simulink library "MultiBodyLibrary"  (R2021b)
settings: Solver=VariableStepAuto  StartTime=0.0  StopTime=10.0  RelTol=1e-3
undefined symbols (not defined in the file or in its folder): gainStruct, useConstraint
libraries: RobotStateLibrary x23, $bdroot x1
settings Model: Creator=icub  LastModifiedBy=icub
settings SolverCC: AlgebraicLoopSolver=TrustRegion
settings DebuggingCC: SFMachineParentedDataDiag=warning

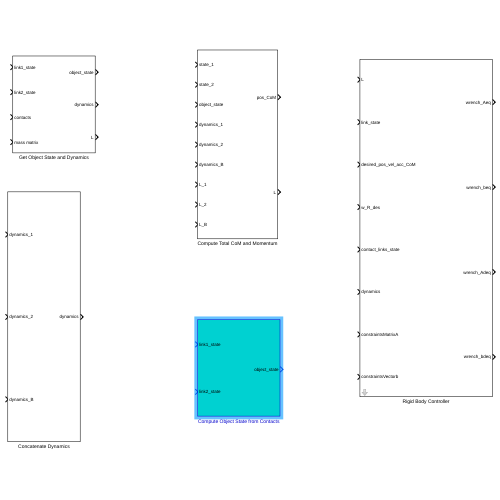
[thumbnail: Simulink's stored preview of the top-level diagram]
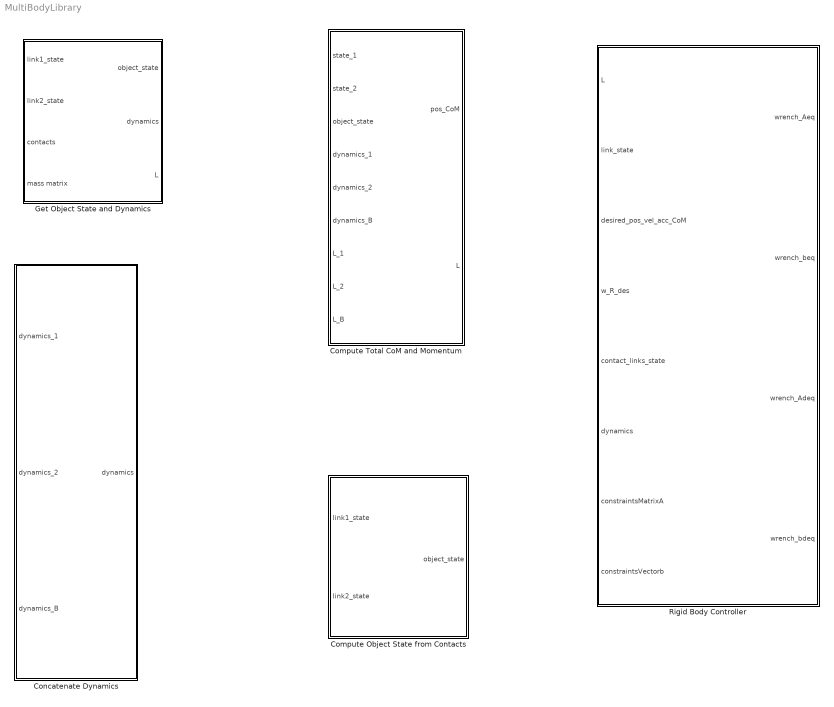
== system MultiBodyLibrary ==
  Compute Object State from Contacts : Subsystem
  Compute Total CoM and Momentum : Subsystem
  Concatenate Dynamics : Subsystem
  Get Object State and Dynamics : Subsystem
  Rigid Body Controller : Subsystem  mask{GainMomentum=gainStruct, linksUseConstraintMatrix=useConstraint}
      mask prompts: GainMomentum "Momentum Control Gain"; linksUseConstraintMatrix "Use Force Constraint on Links"

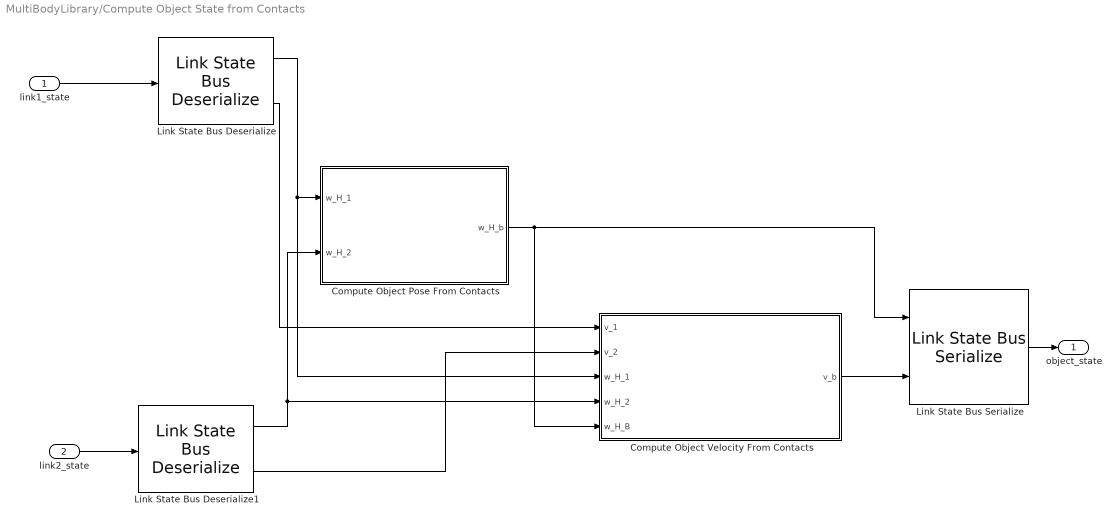
== system MultiBodyLibrary/Compute Object State from Contacts ==
  link1_state : Inport
  link2_state : Inport  Port=2
  Compute Object Pose From Contacts : Subsystem
  Compute Object Velocity From Contacts : Subsystem
  Link State Bus Deserialize : RobotStateLibrary/Link State Bus Deserialize  SystemSampleTime=-1  VariantActivationTime=update diagram  Latency=0  AutoFrameSizeCalculation=off
      settings: SourceProductName=robot-state-library
  Link State Bus Deserialize1 : RobotStateLibrary/Link State Bus Deserialize  SystemSampleTime=-1  VariantActivationTime=update diagram  Latency=0  AutoFrameSizeCalculation=off
      settings: SourceProductName=robot-state-library
  Link State Bus Serialize : RobotStateLibrary/Link State Bus Serialize  SystemSampleTime=-1  VariantActivationTime=update diagram  Latency=0  AutoFrameSizeCalculation=off
      settings: SourceProductName=robot-state-library
  object_state : Outport
  wires:
  Link State Bus Deserialize/1 -> Compute Object Velocity From Contacts/3(w_H_1), Compute Object Pose From Contacts/1(w_H_1)
  Link State Bus Deserialize/2 -> Compute Object Velocity From Contacts/1(v_1)
  Link State Bus Deserialize1/2 -> Compute Object Velocity From Contacts/2(v_2)
  Link State Bus Deserialize1/1 -> Compute Object Velocity From Contacts/4(w_H_2), Compute Object Pose From Contacts/2(w_H_2)
  Compute Object Pose From Contacts/1(w_H_b) -> Link State Bus Serialize/1, Compute Object Velocity From Contacts/5(w_H_B)
  link1_state/1 -> Link State Bus Deserialize/1
  link2_state/1 -> Link State Bus Deserialize1/1
  Compute Object Velocity From Contacts/1(v_b) -> Link State Bus Serialize/2
  Link State Bus Serialize/1 -> object_state/1

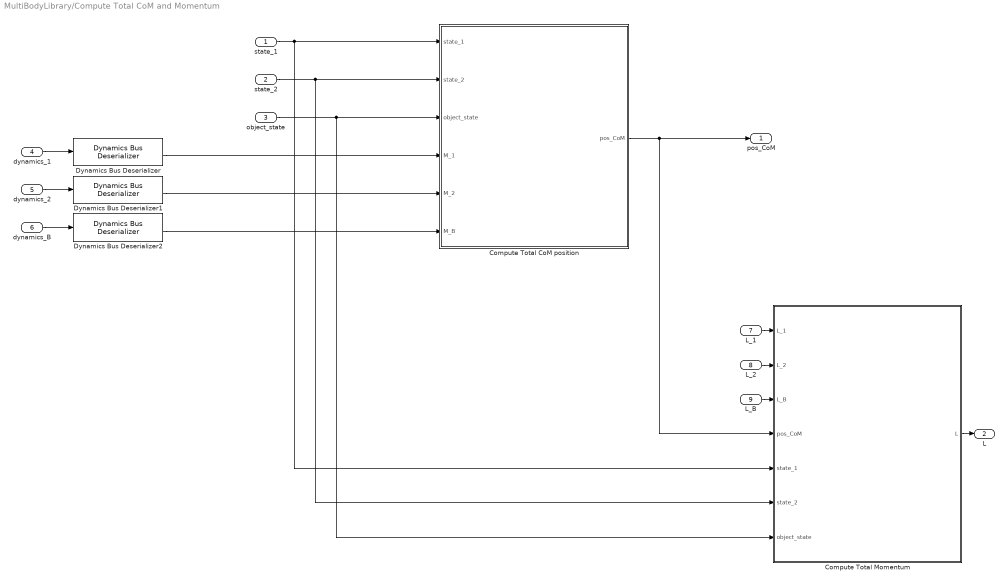
== system MultiBodyLibrary/Compute Total CoM and Momentum ==
  state_1 : Inport
  state_2 : Inport  Port=2
  object_state : Inport  Port=3
  dynamics_1 : Inport  Port=4
  dynamics_2 : Inport  Port=5
  dynamics_B : Inport  Port=6
  L_1 : Inport  Port=7
  L_2 : Inport  Port=8
  L_B : Inport  Port=9
  Compute Total CoM position : Subsystem
  Compute Total Momentum : Subsystem
  Dynamics Bus Deserializer : RobotStateLibrary/Dynamics Bus Deserializer  SystemSampleTime=-1  VariantActivationTime=update diagram  Latency=0  AutoFrameSizeCalculation=off
      settings: SourceProductName=robot-state-library
  Dynamics Bus Deserializer1 : RobotStateLibrary/Dynamics Bus Deserializer  SystemSampleTime=-1  VariantActivationTime=update diagram  Latency=0  AutoFrameSizeCalculation=off
      settings: SourceProductName=robot-state-library
  Dynamics Bus Deserializer2 : RobotStateLibrary/Dynamics Bus Deserializer  SystemSampleTime=-1  VariantActivationTime=update diagram  Latency=0  AutoFrameSizeCalculation=off
      settings: SourceProductName=robot-state-library
  pos_CoM : Outport
  L : Outport  Port=2
  wires:
  L_B/1 -> Compute Total Momentum/3(L_B)
  L_2/1 -> Compute Total Momentum/2(L_2)
  object_state/1 -> Compute Total Momentum/7(object_state), Compute Total CoM position/3(object_state)
  L_1/1 -> Compute Total Momentum/1(L_1)
  Compute Total CoM position/1(pos_CoM) -> Compute Total Momentum/4(pos_CoM), pos_CoM/1
  state_1/1 -> Compute Total Momentum/5(state_1), Compute Total CoM position/1(state_1)
  Compute Total Momentum/1(L) -> L/1
  state_2/1 -> Compute Total Momentum/6(state_2), Compute Total CoM position/2(state_2)
  Dynamics Bus Deserializer/3 -> Compute Total CoM position/4(M_1)
  dynamics_1/1 -> Dynamics Bus Deserializer/1
  dynamics_2/1 -> Dynamics Bus Deserializer1/1
  Dynamics Bus Deserializer1/3 -> Compute Total CoM position/5(M_2)
  Dynamics Bus Deserializer2/3 -> Compute Total CoM position/6(M_B)
  dynamics_B/1 -> Dynamics Bus Deserializer2/1

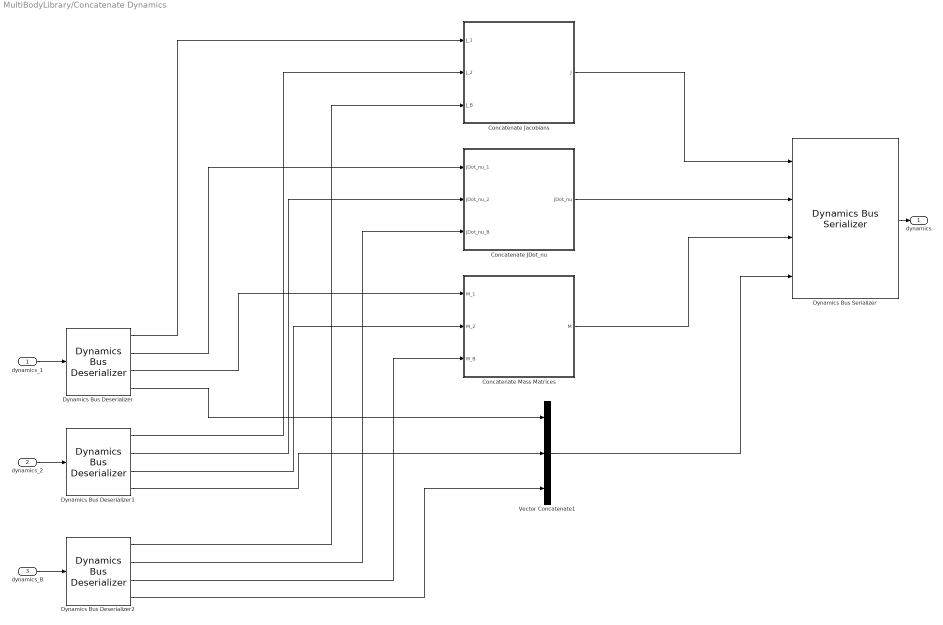
== system MultiBodyLibrary/Concatenate Dynamics ==
  dynamics_1 : Inport
  dynamics_2 : Inport  Port=2
  dynamics_B : Inport  Port=3
  Concatenate JDot_nu : MATLAB Function  TreatAsAtomicUnit=on
  Concatenate Jacobians : MATLAB Function  TreatAsAtomicUnit=on
  Concatenate Mass Matrices : MATLAB Function  TreatAsAtomicUnit=on
  Dynamics Bus Deserializer : RobotStateLibrary/Dynamics Bus Deserializer  SystemSampleTime=-1  VariantActivationTime=update diagram  Latency=0  AutoFrameSizeCalculation=off
      settings: SourceProductName=robot-state-library
  Dynamics Bus Deserializer1 : RobotStateLibrary/Dynamics Bus Deserializer  SystemSampleTime=-1  VariantActivationTime=update diagram  Latency=0  AutoFrameSizeCalculation=off
      settings: SourceProductName=robot-state-library
  Dynamics Bus Deserializer2 : RobotStateLibrary/Dynamics Bus Deserializer  SystemSampleTime=-1  VariantActivationTime=update diagram  Latency=0  AutoFrameSizeCalculation=off
      settings: SourceProductName=robot-state-library
  Dynamics Bus Serializer : RobotStateLibrary/Dynamics Bus Serializer  SystemSampleTime=-1  VariantActivationTime=update diagram  Latency=0  AutoFrameSizeCalculation=off
      settings: SourceProductName=robot-state-library
  Vector Concatenate1 : Concatenate  NumInputs=3
  dynamics : Outport
  wires:
  Dynamics Bus Serializer/1 -> dynamics/1
  Dynamics Bus Deserializer2/4 -> Vector Concatenate1/3
  Concatenate Mass Matrices/1(M) -> Dynamics Bus Serializer/3
  Concatenate Jacobians/1(J) -> Dynamics Bus Serializer/1
  Dynamics Bus Deserializer1/4 -> Vector Concatenate1/2
  Vector Concatenate1/1 -> Dynamics Bus Serializer/4
  Concatenate JDot_nu/1(JDot_nu) -> Dynamics Bus Serializer/2
  Dynamics Bus Deserializer/4 -> Vector Concatenate1/1
  dynamics_1/1 -> Dynamics Bus Deserializer/1
  dynamics_2/1 -> Dynamics Bus Deserializer1/1
  dynamics_B/1 -> Dynamics Bus Deserializer2/1
  Dynamics Bus Deserializer/1 -> Concatenate Jacobians/1(J_1)
  Dynamics Bus Deserializer1/1 -> Concatenate Jacobians/2(J_2)
  Dynamics Bus Deserializer2/1 -> Concatenate Jacobians/3(J_B)
  Dynamics Bus Deserializer/2 -> Concatenate JDot_nu/1(JDot_nu_1)
  Dynamics Bus Deserializer1/2 -> Concatenate JDot_nu/2(JDot_nu_2)
  Dynamics Bus Deserializer2/2 -> Concatenate JDot_nu/3(JDot_nu_B)
  Dynamics Bus Deserializer/3 -> Concatenate Mass Matrices/1(M_1)
  Dynamics Bus Deserializer1/3 -> Concatenate Mass Matrices/2(M_2)
  Dynamics Bus Deserializer2/3 -> Concatenate Mass Matrices/3(M_B)

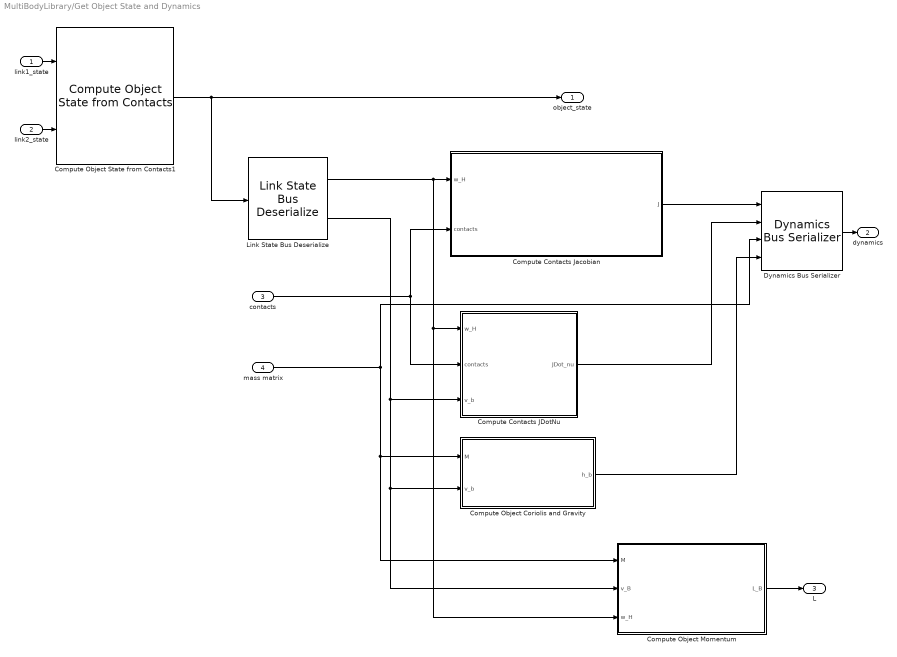
== system MultiBodyLibrary/Get Object State and Dynamics ==
  link1_state : Inport
  link2_state : Inport  Port=2
  contacts : Inport  Port=3
  mass matrix : Inport  Port=4
  Compute Contacts JDotNu : MATLAB Function  TreatAsAtomicUnit=on
  Compute Contacts Jacobian : MATLAB Function  TreatAsAtomicUnit=on
  Compute Object Coriolis and Gravity : MATLAB Function  TreatAsAtomicUnit=on
  Compute Object Momentum : MATLAB Function  TreatAsAtomicUnit=on
  Compute Object State from Contacts1 : $bdroot/Compute Object State from Contacts  SystemSampleTime=-1  VariantActivationTime=update diagram  Latency=0  AutoFrameSizeCalculation=off
  Dynamics Bus Serializer : RobotStateLibrary/Dynamics Bus Serializer  SystemSampleTime=-1  VariantActivationTime=update diagram  Latency=0  AutoFrameSizeCalculation=off
      settings: SourceProductName=robot-state-library
  Link State Bus Deserialize : RobotStateLibrary/Link State Bus Deserialize  SystemSampleTime=-1  VariantActivationTime=update diagram  Latency=0  AutoFrameSizeCalculation=off
      settings: SourceProductName=robot-state-library
  object_state : Outport
  dynamics : Outport  Port=2
  L : Outport  Port=3
  wires:
  link2_state/1 -> Compute Object State from Contacts1/2
  Compute Object State from Contacts1/1 -> Link State Bus Deserialize/1, object_state/1
  link1_state/1 -> Compute Object State from Contacts1/1
  contacts/1 -> Compute Contacts JDotNu/2(contacts), Compute Contacts Jacobian/2(contacts)
  mass matrix/1 -> Compute Object Momentum/1(M), Compute Object Coriolis and Gravity/1(M), Dynamics Bus Serializer/3
  Link State Bus Deserialize/1 -> Compute Object Momentum/3(w_H), Compute Contacts JDotNu/1(w_H), Compute Contacts Jacobian/1(w_H)
  Link State Bus Deserialize/2 -> Compute Object Momentum/2(v_B), Compute Object Coriolis and Gravity/2(v_b), Compute Contacts JDotNu/3(v_b)
  Compute Contacts Jacobian/1(J) -> Dynamics Bus Serializer/1
  Compute Contacts JDotNu/1(JDot_nu) -> Dynamics Bus Serializer/2
  Compute Object Coriolis and Gravity/1(h_b) -> Dynamics Bus Serializer/4
  Dynamics Bus Serializer/1 -> dynamics/1
  Compute Object Momentum/1(L_B) -> L/1

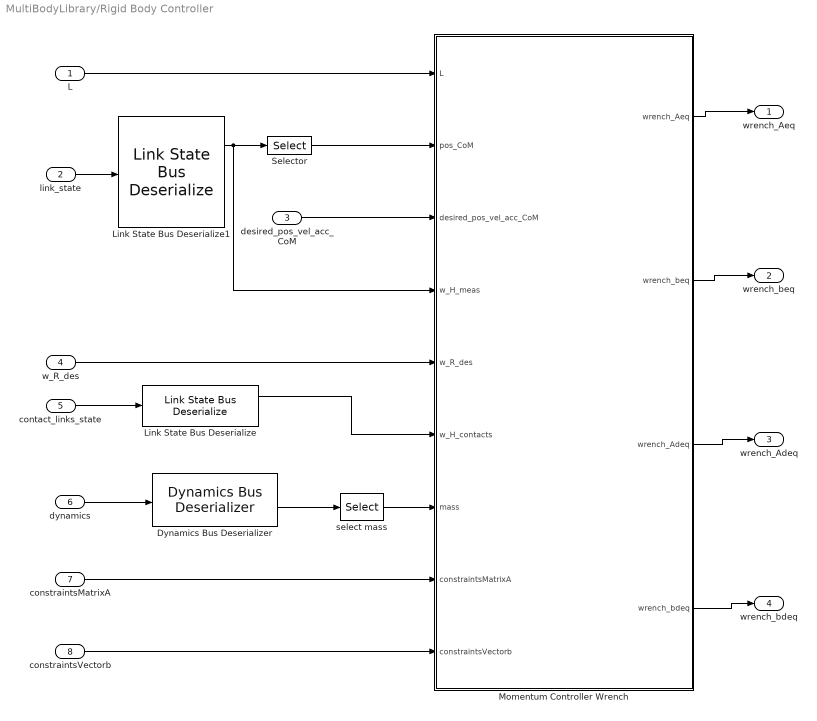
== system MultiBodyLibrary/Rigid Body Controller ==
  L : Inport
  link_state : Inport  Port=2
  desired_pos_vel_acc_CoM : Inport  Port=3
  w_R_des : Inport  Port=4
  contact_links_state : Inport  Port=5
  dynamics : Inport  Port=6
  constraintsMatrixA : Inport  Port=7
  constraintsVectorb : Inport  Port=8
  Dynamics Bus Deserializer : RobotStateLibrary/Dynamics Bus Deserializer  SystemSampleTime=-1  VariantActivationTime=update diagram  Latency=0  AutoFrameSizeCalculation=off
      settings: SourceProductName=robot-state-library
  Link State Bus Deserialize : RobotStateLibrary/Link State Bus Deserialize  SystemSampleTime=-1  VariantActivationTime=update diagram  Latency=0  AutoFrameSizeCalculation=off
      settings: SourceProductName=robot-state-library
  Link State Bus Deserialize1 : RobotStateLibrary/Link State Bus Deserialize  SystemSampleTime=-1  VariantActivationTime=update diagram  Latency=0  AutoFrameSizeCalculation=off
      settings: SourceProductName=robot-state-library
  Momentum Controller Wrench : MATLAB Function  TreatAsAtomicUnit=on
  Selector : Selector  NumberOfDimensions=2  InputPortWidth=3  IndexOptions=Index vector (dialog),Index vector (dialog)  Indices=[1 2 3],4  OutputSizes=1,1
  select mass : Selector  NumberOfDimensions=2  InputPortWidth=3  IndexOptions=Index vector (dialog),Index vector (dialog)  Indices=1,1  OutputSizes=1,1
  wrench_Aeq : Outport
  wrench_beq : Outport  Port=2
  wrench_Adeq : Outport  Port=3
  wrench_bdeq : Outport  Port=4
  wires:
  Momentum Controller Wrench/2(wrench_beq) -> wrench_beq/1
  Momentum Controller Wrench/1(wrench_Aeq) -> wrench_Aeq/1
  Momentum Controller Wrench/3(wrench_Adeq) -> wrench_Adeq/1
  Momentum Controller Wrench/4(wrench_bdeq) -> wrench_bdeq/1
  L/1 -> Momentum Controller Wrench/1(L)
  desired_pos_vel_acc_CoM/1 -> Momentum Controller Wrench/3(desired_pos_vel_acc_CoM)
  constraintsMatrixA/1 -> Momentum Controller Wrench/8(constraintsMatrixA)
  constraintsVectorb/1 -> Momentum Controller Wrench/9(constraintsVectorb)
  link_state/1 -> Link State Bus Deserialize1/1
  Link State Bus Deserialize1/1 -> Momentum Controller Wrench/4(w_H_meas), Selector/1
  contact_links_state/1 -> Link State Bus Deserialize/1
  select mass/1 -> Momentum Controller Wrench/7(mass)
  dynamics/1 -> Dynamics Bus Deserializer/1
  Dynamics Bus Deserializer/3 -> select mass/1
  Selector/1 -> Momentum Controller Wrench/2(pos_CoM)
  Link State Bus Deserialize/1 -> Momentum Controller Wrench/6(w_H_contacts)
  w_R_des/1 -> Momentum Controller Wrench/5(w_R_des)

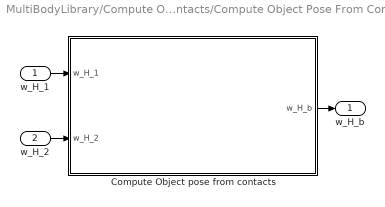
== system MultiBodyLibrary/Compute Object State from Contacts/Compute Object Pose From Contacts ==
  w_H_1 : Inport
  w_H_2 : Inport  Port=2
  Compute Object pose from contacts : MATLAB Function  TreatAsAtomicUnit=on
  w_H_b : Outport
  wires:
  w_H_2/1 -> Compute Object pose from contacts/2(w_H_2)
  Compute Object pose from contacts/1(w_H_b) -> w_H_b/1
  w_H_1/1 -> Compute Object pose from contacts/1(w_H_1)

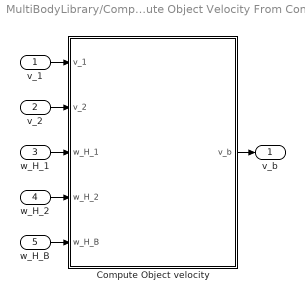
== system MultiBodyLibrary/Compute Object State from Contacts/Compute Object Velocity From Contacts ==
  v_1 : Inport
  v_2 : Inport  Port=2
  w_H_1 : Inport  Port=3
  w_H_2 : Inport  Port=4
  w_H_B : Inport  Port=5
  Compute Object velocity : MATLAB Function  TreatAsAtomicUnit=on
  v_b : Outport
  wires:
  w_H_1/1 -> Compute Object velocity/3(w_H_1)
  w_H_2/1 -> Compute Object velocity/4(w_H_2)
  w_H_B/1 -> Compute Object velocity/5(w_H_B)
  v_1/1 -> Compute Object velocity/1(v_1)
  v_2/1 -> Compute Object velocity/2(v_2)
  Compute Object velocity/1(v_b) -> v_b/1

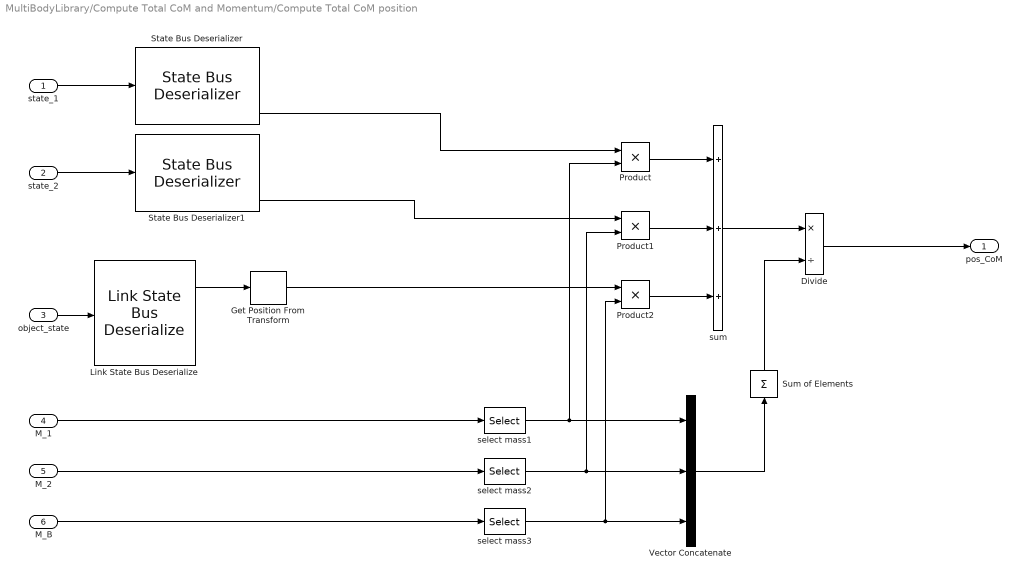
== system MultiBodyLibrary/Compute Total CoM and Momentum/Compute Total CoM position ==
  state_1 : Inport
  state_2 : Inport  Port=2
  object_state : Inport  Port=3
  M_1 : Inport  Port=4
  M_2 : Inport  Port=5
  M_B : Inport  Port=6
  Divide : Product  Inputs=*/
  Get Position From Transform : RobotStateLibrary/Get Position From Transform  SystemSampleTime=-1  VariantActivationTime=update diagram  Latency=0  AutoFrameSizeCalculation=off
      settings: SourceProductName=robot-state-library
  Link State Bus Deserialize : RobotStateLibrary/Link State Bus Deserialize  SystemSampleTime=-1  VariantActivationTime=update diagram  Latency=0  AutoFrameSizeCalculation=off
      settings: SourceProductName=robot-state-library
  Product : Product
  Product1 : Product
  Product2 : Product
  State Bus Deserializer : RobotStateLibrary/State Bus Deserializer  SystemSampleTime=-1  VariantActivationTime=update diagram  Latency=0  AutoFrameSizeCalculation=off
      settings: SourceProductName=robot-state-library
  State Bus Deserializer1 : RobotStateLibrary/State Bus Deserializer  SystemSampleTime=-1  VariantActivationTime=update diagram  Latency=0  AutoFrameSizeCalculation=off
      settings: SourceProductName=robot-state-library
  Sum of Elements : Sum  Inputs=+
  Vector Concatenate : Concatenate  NumInputs=3
  select mass1 : Selector  NumberOfDimensions=2  InputPortWidth=3  IndexOptions=Index vector (dialog),Index vector (dialog)  Indices=1,1  OutputSizes=1,1
  select mass2 : Selector  NumberOfDimensions=2  InputPortWidth=3  IndexOptions=Index vector (dialog),Index vector (dialog)  Indices=1,1  OutputSizes=1,1
  select mass3 : Selector  NumberOfDimensions=2  InputPortWidth=3  IndexOptions=Index vector (dialog),Index vector (dialog)  Indices=1,1  OutputSizes=1,1
  sum : Sum  Inputs=+++
  pos_CoM : Outport  VectorParamsAs1DForOutWhenUnconnected=off
  wires:
  M_B/1 -> select mass3/1
  Product1/1 -> sum/2
  sum/1 -> Divide/1
  select mass2/1 -> Vector Concatenate/2, Product1/2
  Product2/1 -> sum/3
  select mass3/1 -> Vector Concatenate/3, Product2/2
  M_1/1 -> select mass1/1
  select mass1/1 -> Vector Concatenate/1, Product/2
  Vector Concatenate/1 -> Sum of Elements/1
  Divide/1 -> pos_CoM/1
  M_2/1 -> select mass2/1
  Product/1 -> sum/1
  Sum of Elements/1 -> Divide/2
  state_1/1 -> State Bus Deserializer/1
  State Bus Deserializer/4 -> Product/1
  state_2/1 -> State Bus Deserializer1/1
  State Bus Deserializer1/4 -> Product1/1
  Get Position From Transform/1 -> Product2/1
  object_state/1 -> Link State Bus Deserialize/1
  Link State Bus Deserialize/1 -> Get Position From Transform/1

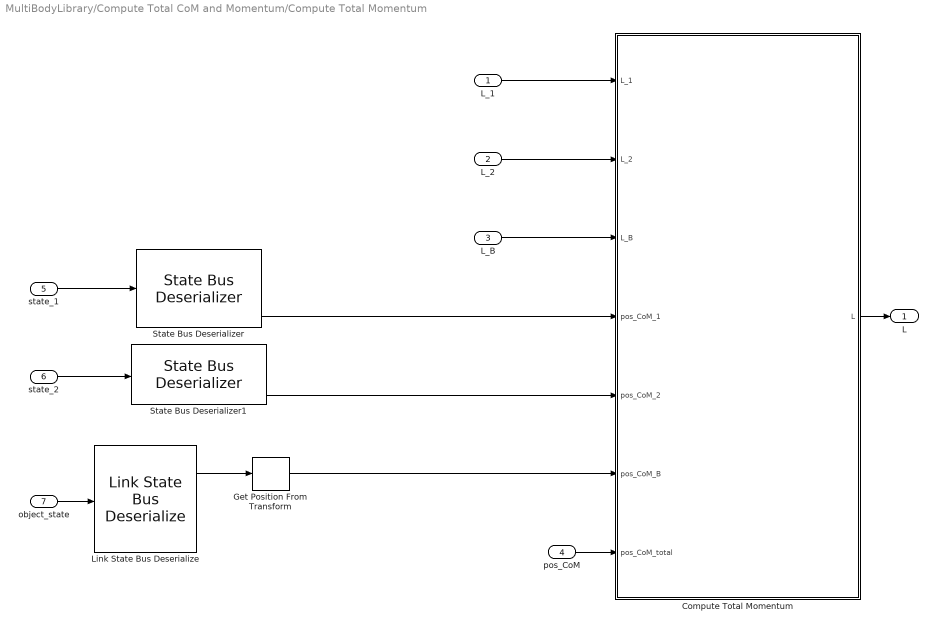
== system MultiBodyLibrary/Compute Total CoM and Momentum/Compute Total Momentum ==
  L_1 : Inport
  L_2 : Inport  Port=2
  L_B : Inport  Port=3
  pos_CoM : Inport  Port=4
  state_1 : Inport  Port=5
  state_2 : Inport  Port=6
  object_state : Inport  Port=7
  Compute Total Momentum : MATLAB Function  TreatAsAtomicUnit=on
  Get Position From Transform : RobotStateLibrary/Get Position From Transform  SystemSampleTime=-1  VariantActivationTime=update diagram  Latency=0  AutoFrameSizeCalculation=off
      settings: SourceProductName=robot-state-library
  Link State Bus Deserialize : RobotStateLibrary/Link State Bus Deserialize  SystemSampleTime=-1  VariantActivationTime=update diagram  Latency=0  AutoFrameSizeCalculation=off
      settings: SourceProductName=robot-state-library
  State Bus Deserializer : RobotStateLibrary/State Bus Deserializer  SystemSampleTime=-1  VariantActivationTime=update diagram  Latency=0  AutoFrameSizeCalculation=off
      settings: SourceProductName=robot-state-library
  State Bus Deserializer1 : RobotStateLibrary/State Bus Deserializer  SystemSampleTime=-1  VariantActivationTime=update diagram  Latency=0  AutoFrameSizeCalculation=off
      settings: SourceProductName=robot-state-library
  L : Outport
  wires:
  L_2/1 -> Compute Total Momentum/2(L_2)
  pos_CoM/1 -> Compute Total Momentum/7(pos_CoM_total)
  L_B/1 -> Compute Total Momentum/3(L_B)
  L_1/1 -> Compute Total Momentum/1(L_1)
  State Bus Deserializer/4 -> Compute Total Momentum/4(pos_CoM_1)
  State Bus Deserializer1/4 -> Compute Total Momentum/5(pos_CoM_2)
  Compute Total Momentum/1(L) -> L/1
  object_state/1 -> Link State Bus Deserialize/1
  state_1/1 -> State Bus Deserializer/1
  Link State Bus Deserialize/1 -> Get Position From Transform/1
  state_2/1 -> State Bus Deserializer1/1
  Get Position From Transform/1 -> Compute Total Momentum/6(pos_CoM_B)

== matlab function MultiBodyLibrary/Concatenate Dynamics/Concatenate Jacobians ==
  data: J_1 input; J output; J_2 input; J_B input
function J = concatenateJacobiansFCN(J_1, J_2, J_B)

J = mbl.concatenateJacobians(J_1, J_2, J_B);

end

== matlab function MultiBodyLibrary/Get Object State and Dynamics/Compute Contacts Jacobian ==
  data: w_H input; J output; contacts input
function J = computeContactsJacobianFCN(w_H, contacts)

J = mbl.computeContactsJacobian(w_H, contacts);

end

== matlab function MultiBodyLibrary/Get Object State and Dynamics/Compute Object Coriolis and Gravity ==
  data: M input; v_b input; h_b output
function h_b = computeObjectCoriolisAndGravityFCN(M, v_b)

h_b = mbl.computeObjectCoriolisAndGravity(M, v_b);

end

== matlab function MultiBodyLibrary/Get Object State and Dynamics/Compute Contacts JDotNu ==
  data: w_H input; JDot_nu output; contacts input; v_b input
function JDot_nu = computeContactsJDotNuFCN(w_H, contacts, v_b)

JDot_nu = mbl.computeContactsJDotNu(w_H, contacts, v_b);

end

== matlab function MultiBodyLibrary/Concatenate Dynamics/Concatenate JDot_nu ==
  data: JDot_nu_1 input; JDot_nu output; JDot_nu_2 input; JDot_nu_B input
function JDot_nu = concatenateJDot_nuFCN(JDot_nu_1, JDot_nu_2, JDot_nu_B)

JDot_nu = mbl.concatenateJDot_nu(JDot_nu_1, JDot_nu_2, JDot_nu_B);

end

== matlab function MultiBodyLibrary/Get Object State and Dynamics/Compute Object Momentum ==
  data: M input; L_B output; v_B input; w_H input
function L_B = computeObjectMomentumInWorldFCN(M, v_B, w_H)

L_B = mbl.computeObjectMomentumInWorld(M, v_B, w_H);

end

== matlab function MultiBodyLibrary/Rigid Body Controller/Momentum Controller Wrench ==
  data: L input; pos_CoM input; desired_pos_vel_acc_CoM input; w_H_meas input; w_R_des input; w_H_contacts input; mass input; wrench_Aeq output; wrench_beq output; wrench_Adeq output; wrench_bdeq output; constraintsMatrixA input; constraintsVectorb input; linksUseConstraintMatrix parameter; GainMomentum parameter
function [wrench_Aeq, wrench_beq, wrench_Adeq, wrench_bdeq] =  momentumControllerWrenchFCN(L, pos_CoM, desired_pos_vel_acc_CoM, w_H_meas, w_R_des, w_H_contacts, mass, constraintsMatrixA, constraintsVectorb, linksUseConstraintMatrix, GainMomentum)

[wrench_Aeq, wrench_beq, wrench_Adeq, wrench_bdeq] = rsl.momentumControllerWrench(L, pos_CoM, desired_pos_vel_acc_CoM, w_H_meas, w_R_des, w_H_contacts, mass, constraintsMatrixA, constraintsVectorb, linksUseConstraintMatrix, GainMomentum);

end

== matlab function MultiBodyLibrary/Concatenate Dynamics/Concatenate Mass Matrices ==
  data: M_1 input; M output; M_2 input; M_B input
function M = concatenateMassMatricesFCN(M_1, M_2, M_B)

M = mbl.concatenateMassMatrices(M_1, M_2, M_B);

end

== matlab function MultiBodyLibrary/Compute Object State from Contacts/Compute Object Pose From Contacts/Compute Object pose from contacts ==
  data: w_H_1 input; w_H_b output; w_H_2 input
function w_H_b = computeObjectPoseFromContactsFCN(w_H_1, w_H_2)

w_H_b = mbl.computeObjectPoseFromContacts(w_H_1, w_H_2, true, false);

end

== matlab function MultiBodyLibrary/Compute Object State from Contacts/Compute Object Velocity From Contacts/Compute Object velocity ==
  data: v_1 input; v_b output; v_2 input; w_H_1 input; w_H_2 input; w_H_B input
function v_b = computeObjectVelocityFromContactsFCN(v_1, v_2, w_H_1, w_H_2, w_H_B)

v_b = mbl.computeObjectVelocityFromContacts(v_1, v_2, w_H_1, w_H_2, w_H_B);

end

== matlab function MultiBodyLibrary/Compute Total CoM and Momentum/Compute Total Momentum/Compute Total Momentum ==
  data: L_1 input; L output; L_2 input; L_B input; pos_CoM_1 input; pos_CoM_2 input; pos_CoM_B input; pos_CoM_total input
function L = computeTotalMomentumFCN(L_1, L_2, L_B, pos_CoM_1, pos_CoM_2, pos_CoM_B, pos_CoM_total)

L = mbl.computeTotalMomentum(L_1, L_2, L_B, pos_CoM_1, pos_CoM_2, pos_CoM_B, pos_CoM_total);

end
